simulink model "VehicleModel"  (R2016b)
settings: Solver=FixedStepAuto  StartTime=0.0  StopTime=t_EndSimulation  FixedStep=base_dT  MaxStep=0.01  RelTol=1e-3  EnableMultiTasking=on
values from neighbouring files (symbols this model uses):
  b_E2C_inloop = Simulink.Parameter    [VehicleModelInit.m]
  b_Engine_in_loop = Simulink.Parameter    [VehicleModelInit.m]
  b_initialize_distance_t_startsim = Simulink.Parameter    [VehicleModelInit.m]
  b_Ne_in_loop = Simulink.Parameter    [VehicleModelInit.m]
  b_TTB_in_loop = Simulink.Parameter    [VehicleModelInit.m]
  b_use_acc = Simulink.Parameter    [VehicleModelInit.m]
  b_use_acc_hardset = Simulink.Parameter    [VehicleModelInit.m]
  base_dT = Simulink.Parameter    [VehicleModelInit.m]
  c_acc_d_hdw = Simulink.Parameter    [VehicleModelInit.m]
  c_acc_hdw = Simulink.Parameter    [VehicleModelInit.m]
  c_EngFricCoef = PARS.c_EngFricCoef    [VehicleModelInit.m]
  c_EngFricCoefd = PARS.c_EngFricCoefd    [VehicleModelInit.m]
  d_Ne_max = Simulink.Parameter    [VehicleModelInit.m]
  d_Ne_min = Simulink.Parameter    [VehicleModelInit.m]
  Driver_TuneG1 = PARS.Driver_TuneG1    [VehicleModelInit.m]
  Driver_TuneG2 = PARS.Driver_TuneG2    [VehicleModelInit.m]
  Driver_TuneG3 = PARS.Driver_TuneG3    [VehicleModelInit.m]
  Driver_TuneG_aw = PARS.Driver_TuneG_aw    [VehicleModelInit.m]
  E2C_c2_dTB = Simulink.Parameter    [VehicleModelInit.m]
  E2C_c_dTB = Simulink.Parameter    [VehicleModelInit.m]
  E2C_CycleTimespan = Simulink.Parameter    [VehicleModelInit.m]
  E2C_initializeRelDist = Simulink.Parameter    [VehicleModelInit.m]
  E2C_SpeedShape = Simulink.Parameter    [VehicleModelInit.m]
  E2C_Trap_CycleAcceEndAlpha = Simulink.Parameter    [VehicleModelInit.m]
  E2C_Trap_CycleAcceStartAlpha = Simulink.Parameter    [VehicleModelInit.m]
  E2C_Trap_CycleDeceEndAlpha = Simulink.Parameter    [VehicleModelInit.m]
  E2C_Trap_CycleDeceStartAlpha = Simulink.Parameter    [VehicleModelInit.m]
  E2C_V_High_kmh = Simulink.Parameter    [VehicleModelInit.m]
  E2C_V_Low_kmh = Simulink.Parameter    [VehicleModelInit.m]
  E2C_V_max = Simulink.Parameter    [VehicleModelInit.m]
  E2C_V_min = Simulink.Parameter    [VehicleModelInit.m]
  FTP_speed_1sec = [FTP_speed_once.speed;Idle_speed_once;FTP_speed_once.speed;Idle_speed_once;FTP_speed_once.speed]    [VehicleModelInit.m]
  mass = 3123*1.3    (= 4059.9)    [VehicleModelInit.m]
  T_ACC_TuneG1_data = Simulink.Parameter    [VehicleModelInit.m]
  T_ACC_TuneG1_pt = Simulink.Parameter    [VehicleModelInit.m]
  T_ACC_TuneG2_data = Simulink.Parameter    [VehicleModelInit.m]
  T_ACC_TuneG2_pt = Simulink.Parameter    [VehicleModelInit.m]
  t_StartSimulation = Simulink.Parameter    [VehicleModelInit.m]
  T_TB_ego_ini = Simulink.Parameter    [VehicleModelInit.m]
  T_TB_OffSet = Simulink.Parameter    [VehicleModelInit.m]
  tau_EngTorque = Simulink.Parameter    [VehicleModelInit.m]
  tau_Ne = Simulink.Parameter    [VehicleModelInit.m]
  tau_pedal_dem = Simulink.Parameter    [VehicleModelInit.m]
  VESP_MD = x0.VESP    [VehicleModelInit.m]
undefined symbols (not defined in the file or in its folder): Continuous, DiscIntNeverNeededParam, initializeRelDist, p_ego_ini, p_lead_ini, PedalMapMD, r_w, Simulation_dT, spsSampleAndHoldModel, v_lead_ini, x0
libraries: simulink x9, spsEdgeDetectorModel x6, dspsigops x1
(part 3 of 7)

== matlab function VehicleModel/Subsystem/Follower vehicle Subsystem/Follow Vehicle/Engine DYnamics and Torque converter ==
  data: time_now input; time_start input; d_Ne output; Ne_rpm input; VSpeed input; last_gearlevel input; GearLevel input; F_tract output; EngineTorque input; Simulate_EngineTorque input; outspeed output; w_ratio output; last_p_2_f input; last_d_Ne input; c_EngFricCoef parameter; p_1_e output; p_2_e output; GR output; torque_ratio output; p1e_ratio output; c_EngFricCoefd parameter
% function [d_Ne, F_tract, outspeed, w_ratio] = gearbox_control(time_now, time_start, Ne_rpm, VSpeed, last_gearlevel, GearLevel, EngineTorque, Simulate_EngineTorque, last_p_2_f, c_EngFricCoef)
% function [d_Ne,F_tract,outspeed,w_ratio]  = gearbox_control(Ne_rpm, VSpeed, GearLevel, EngineTorque)
% %#codegen[d_Ne,F_tract,outspeed,w_ratio]
% % Ne_rpm [rpm]
% % VSpeed [m/s]
% % GearLevel [1~6]
% % EngineTorque [Nm]
% % F_tract [N]
% % d_Ne [rpm]
% % d_Ne [rpm]
% p1.e =0;
% p2.e =0;
% p1.f =0;
% p2.f =0;
% % parameters:
% gearRatio = [3.97	2.31	1.51	1.14	0.85	0.67]';
% FR = 3.51;  % checked with Rasoul 0802
% Rw      = 0.41;     % Tire radius [m] changed  % to match engine speed during 200-300s
% effi_trnsmtn = 0.9;  % not the same as before
% J_Eng = 1.53; %  guess. [kg*m^2]
% 
% GR = gearRatio(GearLevel);  
% 
% % ??????? rpm or rad/s?
% % p1.f = Ne_rpm;  % rpm
% % p2.f = VSpeed * 60/2/pi * FR * GR / Rw;  % rpm
% 
% p1.f = 2*pi/60 * Ne_rpm;  % rad/s
% p2.f = VSpeed * FR * GR / Rw;  % rad/s
% 
% 
% 
% if p1.f==0
%     w_ratio = p2.f/0.1;
% else
%     w_ratio = p2.f/p1.f;
% end
% 
% %  convert speed ratio to capacity factor
% thresh1 = 0.99;
% thresh2 = 1.07;
% thresh3 = 0.85;
% a1 = 11;
% a2 = -10.4038;
% a3 = -1.2657862;
% a4 = 0.28137862;
% a5 = 30.9091;
% a6 = 11118.1;
% a7 = 7.22274;
% a8 = -1.10485;
% a9 = -0.102677;
% b1 = 2.1  ;
% b2 = 1.30588 ;
% b3 = 0.99;
% 
% if (w_ratio < thresh1) 
%     kappa = ((a1 + a2 * w_ratio) / (1 + a3 * w_ratio + a4 * w_ratio^2));
% else
%     if (w_ratio < thresh2) 
%         kappa = (a5 + (w_ratio-thresh1)*a6);
%     else
%         kappa = (a7 / (1 + a8 * exp(a9 * w_ratio)));
%     end
% end
% 
% %  convert speed ratio to torque ratio
% if (w_ratio < thresh3) 
%     torque_ratio = (b1 - b2 * w_ratio);
% else
%     torque_ratio = b3;
% end                                                      
%     kappa = kappa/2; % tune the parameters
%     
% 	p1.e = (p1.f/kappa)^2*sign(1-w_ratio);
% 	p2.e = torque_ratio*p1.e;
%     
%     F_tract = p2.e * effi_trnsmtn * GR * FR / Rw; 
% outspeed = p2.f;
%     % EngineTorque - p1.e = J_Eng * d_w_Eng
%     d_Ne = (EngineTorque - p1.e)/J_Eng * 60/2/pi;
% %     if EngineTorque>100
% %         [EngineTorque, p1.e]
% %     end
% end
%%%%%%%%%%%%%%%%%%%%%%%%%%%%%%%%%%%%%%%%%%%%%%%%%

% 
% 
% function [d_Ne,F_tract,outspeed,w_ratio]  = gearbox_control(Ne_rpm, VSpeed, GearLevel, EngineTorque)
% %#codegen
% % Ne_rpm [rpm]
% % VSpeed [m/s]
% % GearLevel [1~6]
% % EngineTorque [Nm]
% % F_tract [N]
% % d_Ne [rpm]
% p1.e =0;
% p2.e =0;
% p1.f =0;
% p2.f =0;
% 
% 
% % parameters:
% gearRatio = [3.97	2.31	1.51	1.14	0.85	0.67]';
% FR = 3.51;  % checked with Rasoul 0802
% Rw      = 0.41;     % Tire radius [m] changed  % to match engine speed during 200-300s
% effi_trnsmtn = 0.9;
% J_Eng = 1.53; %  guess. [kg*m^2]
% 
% GR = gearRatio(GearLevel);  
% 
% % ??????? rpm or rad/s?
% p1.f = Ne_rpm;  % rpm
% p2.f = VSpeed * 60/2/pi * FR * GR / Rw;  % rpm
% 
% p1.f = 2*pi/60 * Ne_rpm;  % rad/s
% p2.f = VSpeed * FR * GR / Rw;  % rad/s
% 
% 
% 
% if p1.f==0
%     w_ratio = p2.f/0.1;
% else
%     w_ratio = p2.f/p1.f;
% end;
% 
% %  convert speed ratio to capacity factor
% % Original Tulga and Xinyi's parameters
% % thresh1 = 0.99;
% % thresh2 = 1.07;
% % thresh3 = 0.85;
% % a1 = 11;
% % a2 = -10.4038;
% % a25 = 0;
% % a3 = -1.2657862;
% % a4 = 0.28137862;
% % a5 = 30.9091;
% % a6 = 11118.1;
% % a7 = 7.22274;
% % a8 = -1.10485;
% % a9 = -0.102677;
% % b1 = 2.1;
% % b2 = 1.30588;
% % b3 = 0.99;
% % TuneRatio = 1;
% 
% % parameters from shape in reference:
% % Nonlinear Robust Control of Torque Converter
% % Clutch Slip System for Passenger Vehicles Using
% % Advanced Torque Estimation Algorithms
% thresh1 = 1;
% thresh2 = 1.07;
% thresh3 = 0.85;
% a1 = 11;
% a2 = -10.4038/1.2;
% a25 = 0;
% a3 = -1.2657862;
% a4 = 0.28137862;
% a5 = 30.9091/43*202;
% a6 = 11118.1;
% a7 = 7.22274*150*2.5/9;
% a8 = -1.10485;
% a9 = -0.102677*4.5;
% b1 = 2.1;
% b2 = 1.30588;
% b3 = 0.99;
% 
% 
% TuneRatio = 2;
% 
% if (w_ratio < thresh1) 
%     kappa = ((a1 + a2 * w_ratio + a25* w_ratio^2) /(1 + a3 * w_ratio + a4 * w_ratio^2));
% else
%     if (w_ratio < thresh2) 
%         kappa = (a5 + (w_ratio-thresh1)*a6);
%     else
%         kappa = 1/sqrt((1/11^2-1/923^2)/4/(1.5-1.07)*(w_ratio-thresh2)+1/923^2);
%         % kappa = (a7 / (1 + a8 * exp(a9 * w_ratio)));
%     end
% end
% kappa = kappa/TuneRatio; % tune the parameters
% %  convert speed ratio to torque ratio
% % 	if (w_ratio < thresh3) 
% % 		torque_ratio = (b1 - b2 * w_ratio);
% % 	else
% % 		torque_ratio = b3;
% %     end                                                     
%     if (w_ratio < thresh3) 
%         torque_ratio = (b1 - b2 * w_ratio);
%     elseif w_ratio >= thresh3 && w_ratio<=1
%         torque_ratio = b3;
%     else
%         torque_ratio = b3 + w_ratio-1;
%     end
% 	p1.e = (p1.f/kappa)^2*sign(1-w_ratio);
% 	p2.e = torque_ratio*p1.e;
%     
%     F_tract = p2.e * effi_trnsmtn * GR * FR / Rw; 
% 
%     % EngineTorque - p1.e = J_Eng * d_w_Eng
%     d_Ne = (EngineTorque - p1.e)/J_Eng * 60/2/pi;
% outspeed = p2.f;
% end
% % 

% %%%%%%%%%%%%%%%%%%%%%%%%%%%%%%%%%%%%%%%%%%%%%%%%%%%%%%
% My original TC:
function [d_Ne,F_tract,outspeed,w_ratio,p_1_e,p_2_e,GR,torque_ratio, p1e_ratio]  = gearbox_control(time_now, time_start, Ne_rpm, VSpeed, last_gearlevel, GearLevel, EngineTorque, Simulate_EngineTorque, last_p_2_f, last_d_Ne, c_EngFricCoef,c_EngFricCoefd)
%#codegen
% Ne_rpm [rpm]
% VSpeed [m/s]
% GearLevel [1~6]
% EngineTorque [Nm]
% F_tract [N]
% d_Ne [rpm]
p1.e =0;
p2.e =0;
p1.f =0;
p2.f =0;


    % parameters:
    gearRatio = [3.97	2.31	1.51	1.14	0.85	0.67]';
    FR = 3.51;  % checked with Rasoul 0802
    Rw      = 0.41;     % Tire radius [m] changed  % to match engine speed during 200-300s
    effi_trnsmtn = 0.9;
    J_Eng = 2.53; % Original value when doing alpha openloop: 1.53; %  guess. [kg*m^2]
    time_duration = [0.7,0.7,0.6,0.5,0.5,0.5] + 0.4;   % 0.5 [s] gear shift duration.
 
    % ---------------------------------------------
    % This part modified based on Tulga's code:
    % ng = gr2 + ((gr1-gr2)/dur)*(time-ts);
    % nt = gr2*eff2 + ((gr1*eff1-gr2*eff2)/dur)*(time-ts);
    
    if time_now < time_start + time_duration(GearLevel)
        ratio = (time_now - time_start)/time_duration(GearLevel);
        GR = gearRatio(GearLevel) * ratio + gearRatio(last_gearlevel) * (1 - ratio);  
        % EngineTorque = Simulate_EngineTorque;  % During shifts, use simulated torque. 
    else
        GR = gearRatio(GearLevel);
    end
    % ---------------------------------------------

    % ??????? rpm or rad/s?
    p1.f = Ne_rpm;  % rpm
    p2.f = VSpeed * 60/2/pi * FR * GR / Rw;  % rpm

    p1.f = 2*pi/60 * Ne_rpm;  % rad/s
    p2.f = VSpeed * FR * GR / Rw;  % rad/s
    % p2.f = max(min(p2.f, last_p_2_f+80*0.02), last_p_2_f-80*0.02); % Removed
    % because already done the smoothing in GR. This line generates similar Ne
    % and slightly less torque than if using linear combination above. 


    if p1.f<=0.1
        w_ratio = p2.f/0.1;
    else
        w_ratio = p2.f/p1.f;
    end
    
    clutch_efficiency = 1;
%     if time_now < time_start + time_duration(GearLevel)
%         clutch_efficiency = w_ratio;
%     else
%         clutch_efficiency = 1;
%     end
    
    %  convert speed ratio to capacity factor

    thresh1 = 1;
    thresh2 = 1.07;
    thresh3 = 0.85;
    a1 = 11.5;
    a2 = -10.4038/1.2;
    a25 = -0.04;
    a3 = -1.2657862;
    a4 = 0.28137862;
    a5 = 30.9091/43*202;
    a6 = 11118.1;
    a7 = 7.22274*150*2.5/9;
    a8 = -1.10485;
    a9 = -0.102677*4.5;
    b1 = 2.1*1.2; % 2.0; % *0.7
    b2 = 1.8; % 3.7765; % 2.5412; % 2.0471; % 1.30588; % 0.5647; % 1.30588 * 0.7;
    b3 = 0.99;
    TuneRatio =2;

% b1 = 1.6;
% b2 = 0.90588;

    if (w_ratio <= thresh1) 
        if  w_ratio >0.5
            % xx=interp1([0.5,0.6,0.7,0.8,0.9,1],[0.9,0.85,0.7,0.6,0.3,0.01],w_ratio,'PCHIP');
            xx=interp1([0.5,0.6,0.7,0.8,0.9,1],[0.85,0.78,0.65,0.5,0.3,0.01],w_ratio,'PCHIP');
            xx = max(xx,0);
            kappa = sqrt(1/xx/0.033)*TuneRatio;

        else
            % xx=interp1([0,0.4,0.5],[1,0.95,0.9],w_ratio,'PCHIP');
            xx=interp1([0,0.4,0.5],[1,0.9,0.85],w_ratio,'PCHIP');
            xx = max(xx,0);
            kappa = sqrt(1/xx/0.033)*TuneRatio;

        end
    else
        if (w_ratio < thresh2) 
            kappa = (a5 + (w_ratio-thresh1)*a6);
        else
            kappa = (1/sqrt((1/11^2-1/923^2)/4/(1.5-1.07)*(w_ratio-thresh2)+1/923^2))*1.0;
            % kappa = ((a7+(exp(w_ratio))^-2-2) / (1 + a8 * exp(a9 * w_ratio)))+1/(10^20*(25*(w_ratio-thresh2)+0.1).^20);
        end
    end

    if (w_ratio < thresh3) 
        torque_ratio = (b1 - b2 * w_ratio);
    elseif (w_ratio >= thresh3) && (w_ratio<=1)
        torque_ratio = b3;
    else
        % torque_ratio = b3 + (w_ratio-1)*2;
        torque_ratio = b3 + (w_ratio-1)*1 + 2*((1-1.5)^2-(w_ratio-1.5)^2);
        % torque_ratio = b3;
        % torque_ratio = b3 + w_ratio-1;
    end
    kappa = kappa/TuneRatio; % tune the parameters

	p1.e = (p1.f/kappa)^2*sign(1-w_ratio);
	p2.e = torque_ratio*p1.e * clutch_efficiency;
    
    F_tract = p2.e * effi_trnsmtn * GR * FR / Rw; 

    % EngineTorque - p1.e = J_Eng * d_w_Eng
    
    d_Ne = (EngineTorque - p1.e - c_EngFricCoef*(Ne_rpm-500) - c_EngFricCoefd*last_d_Ne)/J_Eng * 60/2/pi;
    
    p_1_e = p1.e;
    p_2_e = p2.e;
    
    outspeed = p2.f;
    p1e_ratio = 1/(kappa)^2;
    
end

%%%%%%%%%%%%%%%%%%%%%%%%%%%%%%%%%%%%%%%%%%
% Try Tulga's torque converter
% 
% 
% function [d_Ne,F_tract,outspeed,w_ratio]  = gearbox_control(...
% time_now, time_start, Ne_rpm, VSpeed, last_gearlevel, GearLevel, ...
%     EngineTorque, Simulate_EngineTorque, last_p_2_f, c_EngFricCoef)
%     % Ne_rpm, VSpeed, GearLevel, EngineTorque)
% 
% %#codegen
% % Ne_rpm [rpm]
% % VSpeed [m/s]
% % GearLevel [1~6]
% % EngineTorque [Nm]
% % F_tract [N]
% % d_Ne [rpm]
% p1.e =0;
% p2.e =0;
% p1.f =0;
% p2.f =0;
% 
% 
% % parameters:
% gearRatio = [3.97	2.31	1.51	1.14	0.85	0.67]';
% FR = 3.51;  % checked with Rasoul 0802
% Rw      = 0.41;     % Tire radius [m] changed  % to match engine speed during 200-300s
% effi_trnsmtn = 0.9;
% J_Eng = 1.53; %  guess. [kg*m^2]
% time_duration = [0.7,0.7,0.6,0.5,0.5,0.5] + 0.2;   % 0.5 [s] gear shift duration.
% 
% % GR = gearRatio(GearLevel);  
% if time_now < time_start + time_duration(GearLevel)
%     ratio = (time_now - time_start)/time_duration(GearLevel);
%     GR = gearRatio(GearLevel) * ratio + gearRatio(last_gearlevel) * (1 - ratio);  
%     % EngineTorque = Simulate_EngineTorque;  % During shifts, use simulated torque. 
% else
%     GR = gearRatio(GearLevel);
% end
% 
% 
% % ??????? rpm or rad/s?
% p1.f = Ne_rpm;  % rpm
% p2.f = VSpeed * 60/2/pi * FR * GR / Rw;  % rpm
% 
% p1.f = 2*pi/60 * Ne_rpm;  % rad/s
% p2.f = VSpeed * FR * GR / Rw;  % rad/s
% 
% 
% 
% if p1.f==0
%     w_ratio = p2.f/0.1;
% else
%     w_ratio = p2.f/p1.f;
% end;
% 
% % %  convert speed ratio to capacity factor
% % % Original Tulga and Xinyi's parameters
% % thresh1 = 0.99;
% % thresh2 = 1.07;
% % thresh3 = 0.85;
% % a1 = 11;
% % a2 = -10.4038;
% % a25 = 0;
% % a3 = -1.2657862;
% % a4 = 0.28137862;
% % a5 = 30.9091;
% % a6 = 11118.1;
% % a7 = 7.22274;
% % a8 = -1.10485;
% % a9 = -0.102677;
% % b1 = 2.1;
% % b2 = 1.30588;
% % b3 = 0.99;
% % TuneRatio = 1;
% 
% % parameters from shape in reference:
% % Nonlinear Robust Control of Torque Converter
% % Clutch Slip System for Passenger Vehicles Using
% % Advanced Torque Estimation Algorithms
% thresh1 = 1;
% thresh2 = 1.07;
% thresh3 = 0.85;
% a1 = 11;
% a2 = -10.4038/1.2;
% a25 = 0;
% a3 = -1.2657862;
% a4 = 0.28137862;
% a5 = 30.9091/43*202;
% a6 = 11118.1;
% a7 = 7.22274*150*2.5/9;
% a8 = -1.10485;
% a9 = -0.102677*4.5;
% b1 = 2.1;
% b2 = 1.30588;
% b3 = 0.99;
% % 
% % 
% TuneRatio = 2;
% 
% if (w_ratio < thresh1) 
%     kappa = ((a1 + a2 * w_ratio + a25* w_ratio^2) /(1 + a3 * w_ratio + a4 * w_ratio^2));
% else
%     if (w_ratio < thresh2) 
%         kappa = (a5 + (w_ratio-thresh1)*a6);
%     else
%         kappa = 1/sqrt((1/11^2-1/923^2)/4/(1.5-1.07)*(w_ratio-thresh2)+1/923^2);
%         % kappa = (a7 / (1 + a8 * exp(a9 * w_ratio)));
%     end
% end
% kappa = kappa/TuneRatio; % tune the parameters
% %  convert speed ratio to torque ratio
% % 	if (w_ratio < thresh3) 
% % 		torque_ratio = (b1 - b2 * w_ratio);
% % 	else
% % 		torque_ratio = b3;
% %     end                                                     
%     if (w_ratio < thresh3) 
%         torque_ratio = (b1 - b2 * w_ratio);
%     elseif w_ratio >= thresh3 && w_ratio<=1
%         torque_ratio = b3;
%     else
%         torque_ratio = b3 + w_ratio-1;
%     end
% 	p1.e = (p1.f/kappa)^2*sign(1-w_ratio);
% 	p2.e = torque_ratio*p1.e;
%     
%     F_tract = p2.e * effi_trnsmtn * GR * FR / Rw; 
% 
%     % EngineTorque - p1.e = J_Eng * d_w_Eng
%     d_Ne = (EngineTorque - p1.e)/J_Eng * 60/2/pi;
% outspeed = p2.f;
% end
% %

== matlab function VehicleModel/Subsystem/Follower vehicle Subsystem/Follow Vehicle/PthsetTq model ==
  data: Tq_vec output; Ne_vec input; Torque_vec input; VSpeed_vec input
function Tq_vec    = PthsetModel(Ne_vec, Torque_vec, VSpeed_vec)
%#codegen


FordTqCal.Ne = [500;500;500;500;500;500;500;500;600;600;600;600;600;600;600;600;800;800;800;800;800;800;800;800;800;1000;1000;1000;1000;1000;1000;1000;1000;1000;1000;1200;1200;1200;1200;1200;1200;1200;1200;1200;1200;1200;1400;1400;1400;1400;1400;1400;1400;1400;1400;1400;1400;1400;1400;1400;1600;1600;1600;1600;1600;1600;1600;1600;1600;1600;1600;1600;1600;1600;1600;1600;1800;1800;1800;1800;1800;1800;1800;1800;1800;1800;1800;1800;1800;1800;1800;1800;1800;2000;2000;2000;2000;2000;2000;2000;2000;2000;2000;2000;2000;2000;2000;2000;2000;2000;2200;2200;2200;2200;2200;2200;2200;2200;2200;2200;2200;2200;2200;2200;2200;2200;2200;2400;2400;2400;2400;2400;2400;2400;2400;2400;2400;2400;2400;2400;2400;2400;2400;2400;2600;2600;2600;2600;2600;2600;2600;2600;2600;2600;2600;2600;2600;2600;2600;2600;2600;2800;2800;2800;2800;2800;2800;2800;2800;2800;2800;2800;2800;2800;2800;2800;2800;2800;3000;3000;3000;3000;3000;3000;3000;3000;3000;3000;3000;3000;3000;3000;3000;3000;3200;3200;3200;3200;3200;3200;3200;3200;3200;3200;3200;3200;3200;3200;3200;3400;3400;3400;3400;3400;3400;3400;3400;3400;3400;3400;3400;3400;500;600;800;1000;1200;1400;1600;1800;2000;2200;2400;2600;2800;3000;3200;3400];
FordTqCal.Torque = [-74.9710029200000;-16.8452928900000;22.5768412100000;66.3118405400000;122.485125100000;171.724968200000;209.291492900000;327.216453100000;-69.7798932200000;-17.2465227700000;24.2147953500000;71.9971179100000;108.756652100000;165.981760000000;232.925894200000;339.093048300000;-71.2481971900000;6.78186051200000;38.9692268100000;99.4179257300000;149.909041800000;196.908789400000;242.879963800000;344.770267100000;422.698119600000;-77.1395675800000;2.25202763800000;42.2012448800000;93.5939964800000;136.909750000000;186.449928000000;240.720366800000;341.467734600000;436.725202700000;518.667213700000;-77.8024739700000;-3.56634450800000;41.4527193700000;93.4652855300000;142.232771000000;187.634317800000;236.637760000000;333.810753400000;431.126064600000;524.171115900000;615.577708700000;-83.4754614100000;-8.34883757200000;37.4277251100000;92.8230069100000;140.027350900000;182.326160900000;231.941433200000;328.194558900000;424.562740900000;511.984434000000;616.532564800000;717.468056700000;811.174744000000;854.007744200000;-94.0440471900000;-11.9160323900000;33.5026669500000;81.9477706700000;136.063332400000;181.688248000000;229.433752100000;327.668074700000;421.229442600000;505.624945100000;607.627890900000;702.803483900000;796.506491400000;901.631690000000;1006.15607900000;1167.16171800000;-105.810334300000;-29.5507777900000;26.4565543900000;79.4188075700000;129.112641000000;174.814601000000;227.881676400000;320.856473100000;409.287739500000;498.839210100000;595.698470400000;692.151257500000;782.649266900000;879.386444600000;991.660780600000;1084.17976600000;1166.69977800000;-115.283222900000;-26.7879707200000;30.5205674100000;71.0457994800000;115.255625000000;163.862045400000;213.681720400000;312.680641600000;402.357125500000;491.118597900000;585.701714300000;684.640373900000;777.887954900000;871.133695900000;978.600076500000;1069.07187300000;1159.94140700000;-117.321614400000;-35.7200974500000;13.9601127100000;65.4809546500000;107.970297900000;157.171490300000;206.297887200000;308.097810300000;387.385807300000;489.362517700000;575.402137900000;676.483194500000;768.282516600000;857.450964200000;959.454329600000;1055.35717600000;1161.03658800000;-124.259281100000;-43.0894697100000;9.89302132700000;59.3682431900000;99.0452310000000;149.131037800000;197.173036500000;296.308032200000;373.776023900000;471.134821700000;565.528338100000;659.058943700000;749.259571300000;843.445347900000;945.856414300000;1036.61175100000;1159.60480900000;-135.365963400000;-61.2876489400000;-4.33545738900000;41.0434879000000;90.6662490300000;137.731564000000;186.322276200000;279.595050000000;364.630774700000;457.697283200000;551.990748200000;640.398723700000;730.372979000000;818.138407600000;919.270429500000;1012.50988300000;1144.92866700000;-154.608877100000;-62.4754987700000;-13.0688869200000;35.1175674200000;78.5403251000000;131.062560100000;176.973940900000;267.098275700000;355.041255000000;439.823605800000;530.465621200000;615.923600900000;700.034455300000;789.041537900000;888.954149400000;980.416288500000;1117.56934700000;-166.473853800000;-95.8158145100000;-30.2112397100000;20.7283938700000;66.7200572800000;113.495783000000;162.476945100000;258.772843200000;342.012303800000;426.753454600000;521.939682100000;602.320677600000;682.204738400000;762.344949700000;873.583209600000;992.218131200000;-173.479879900000;-101.615500000000;-50.5548781900000;5.59668278300000;48.8622091200000;99.0922829400000;147.984848200000;232.803380700000;327.097768100000;400.176971300000;486.274910900000;575.903432100000;672.200276300000;766.611653100000;813.925270700000;-177.160793600000;-110.511019900000;-63.6365230300000;-14.9158481100000;30.4639121500000;78.5632367300000;129.668192000000;224.303438100000;301.548553800000;389.638590300000;473.171130000000;566.041266600000;638.739388800000;-1000;-1000;-1000;-1000;-1000;-1000;-1000;-1000;-1000;-1000;-1000;-1000;-1000;-1000;-1000;-1000];
FordTqCal.PthsetTq = [0;50;100;150;200;250;300;400;0;50;100;150;200;250;300;400;0;50;100;150;200;250;300;400;500;0;50;100;150;200;250;300;400;500;600;0;50;100;150;200;250;300;400;500;600;700;0;50;100;150;200;250;300;400;500;600;700;800;900;1000;0;50;100;150;200;250;300;400;500;600;700;800;900;1000;1100;1300;0;50;100;150;200;250;300;400;500;600;700;800;900;1000;1100;1200;1300;0;50;100;150;200;250;300;400;500;600;700;800;900;1000;1100;1200;1300;0;50;100;150;200;250;300;400;500;600;700;800;900;1000;1100;1200;1300;0;50;100;150;200;250;300;400;500;600;700;800;900;1000;1100;1200;1350;0;50;100;150;200;250;300;400;500;600;700;800;900;1000;1100;1200;1350;0;50;100;150;200;250;300;400;500;600;700;800;900;1000;1100;1200;1350;0;50;100;150;200;250;300;400;500;600;700;800;900;1000;1100;1250;0;50;100;150;200;250;300;400;500;600;700;800;900;1000;1050;0;50;100;150;200;250;300;400;500;600;700;800;850;0;0;0;0;0;0;0;0;0;0;0;0;0;0;0;0];

Tq_vec = griddata(FordTqCal.Ne, FordTqCal.Torque, FordTqCal.PthsetTq, Ne_vec, Torque_vec);
Tq_vec( intersect(find(VSpeed_vec<2), find(Torque_vec<5) )) = 150;
Tq_vec( intersect( find(isnan(Tq_vec)), find(Torque_vec<0)) )=0;

== matlab function VehicleModel/Subsystem/Follower vehicle Subsystem/Follow Vehicle/Engine model1 ==
  data: engineoutNOx_ppm output; Ne_vec input; Tq_vec input; meu_kg_s output
function [engineoutNOx_ppm, meu_kg_s]      = EngineModel(Ne_vec, Tq_vec)
%#codegen
FordData.C_NOx_eu=[2.25762409700000,1.48625333300000,2.53227143100000,1.40526886500000,1.48376886900000,1.08211845400000,1.22896117600000,0.774905453000000,1.43134235500000,1.10964119300000,1.16812440600000,0.912941239000000,1.27689041400000,0.840189182000000,1.68537425400000,1.06896694300000;77.7336189200000,66.7131323400000,83.1490420600000,71.4323197300000,78.6699699800000,83.1126174900000,91.0357459700000,80.5169999300000,86.1282940600000,74.9800580500000,77.9368165100000,67.3535086200000,67.6916369000000,52.9319036300000,57.6801792200000,56.9409641600000;93.4701856100000,73.0093723900000,93.1112276200000,63.5327023300000,70.5283689500000,69.8944052300000,69.7843775900000,78.9711420600000,108.102874500000,99.0763243400000,109.785688800000,103.569999900000,111.936107900000,108.116904900000,138.463511700000,161.283675000000;115.900969600000,98.1385357700000,90.1779151700000,75.7649708100000,68.3221778600000,61.6508764000000,80.9472557300000,92.3232953600000,118.429404700000,118.138823600000,125.300058600000,131.164566000000,147.137470100000,152.844180100000,218.902575100000,277.520714200000;244.974877800000,208.876505900000,132.824970000000,97.4586493500000,78.8352280100000,77.3417367800000,108.319940000000,113.631075200000,131.433696700000,141.663772500000,139.357590500000,161.691976400000,176.291578900000,192.054131800000,282.689702500000,409.127621500000;611.801796900000,455.626928300000,203.786423900000,135.014024300000,114.974255700000,105.941999700000,128.123614400000,139.780695500000,174.086505800000,179.955149700000,192.886726200000,211.508862200000,235.443617300000,238.055294500000,360.565449900000,547.683923500000;1331.45555700000,1219.17445500000,456.065104100000,220.679940100000,134.895568700000,124.843727900000,157.453367900000,179.159511200000,246.544523800000,254.239942600000,278.443091200000,283.519117800000,302.382694400000,297.501244000000,453.310748900000,678.719456500000;1689.28144100000,1662.56946000000,1809.85647000000,756.339463100000,279.077382200000,175.138930500000,189.261489800000,223.400363300000,291.671666000000,349.664945600000,388.014190700000,413.407484800000,433.835298400000,420.357427800000,608.756011200000,876.977261900000;1689.28144100000,1662.56946000000,2030.22882400000,2372.79262800000,604.193954500000,305.600904600000,261.407409900000,262.680665700000,349.460689000000,508.980239700000,542.334583100000,560.582959100000,544.666544600000,596.865821800000,773.404254300000,950.574495400000;1689.28144100000,1662.56946000000,2030.22882400000,1903.18924700000,1065.21376900000,549.108273800000,462.245157500000,361.353571400000,486.090349200000,651.363421300000,655.258364400000,676.150537900000,615.765239500000,686.080323600000,847.960568400000,1032.08809900000;1689.28144100000,1662.56946000000,2030.22882400000,1903.18924700000,1838.81377000000,1293.62411500000,766.547606300000,634.774793300000,700.457916600000,738.703189700000,735.874044500000,728.241260300000,678.368811500000,715.053387000000,881.818869800000,1066.88343700000;1689.28144100000,1662.56946000000,2030.22882400000,1903.18924700000,1838.81377000000,1698.37125200000,1142.32010400000,964.476765700000,940.581138700000,877.995809400000,851.089467800000,793.700416400000,780.098073200000,795.836746800000,934.802528500000,1059.46738200000;1689.28144100000,1662.56946000000,2030.22882400000,1903.18924700000,1838.81377000000,1869.57849400000,1747.34970100000,1358.95454200000,1138.71021400000,915.954867900000,899.966250500000,897.467100600000,866.129469200000,837.367378600000,920.021667500000,1031.69091400000;1689.28144100000,1662.56946000000,2030.22882400000,1903.18924700000,1838.81377000000,1759.27605400000,1998.77750900000,1517.83313700000,1276.92765800000,1054.38757200000,908.992011100000,922.976109300000,904.774372800000,833.394516900000,892.743814300000,1031.69091400000;1689.28144100000,1662.56946000000,2030.22882400000,1903.18924700000,1838.81377000000,1759.27605400000,1936.27559700000,1736.12530100000,1538.87784600000,1259.82010600000,1122.27134200000,1040.75706100000,997.544178500000,902.754910600000,897.219403800000,1031.69091400000;1689.28144100000,1662.56946000000,2030.22882400000,1903.18924700000,1838.81377000000,1759.27605400000,1643.64035700000,1776.66432900000,1639.86910900000,1405.51736700000,1269.69058700000,1111.13832700000,979.684554000000,899.367364400000,897.219403800000,1031.69091400000;1689.28144100000,1662.56946000000,2030.22882400000,1903.18924700000,1838.81377000000,1759.27605400000,1643.64035700000,1677.73846200000,1572.58036400000,1358.57810700000,1204.91369200000,1046.82235300000,882.208603300000,899.367364400000,897.219403800000,1031.69091400000];
FordData.spd=[500,600,800,1000,1200,1400,1600,1800,2000,2200,2400,2600,2800,3000,3200,3400;500,600,800,1000,1200,1400,1600,1800,2000,2200,2400,2600,2800,3000,3200,3400;500,600,800,1000,1200,1400,1600,1800,2000,2200,2400,2600,2800,3000,3200,3400;500,600,800,1000,1200,1400,1600,1800,2000,2200,2400,2600,2800,3000,3200,3400;500,600,800,1000,1200,1400,1600,1800,2000,2200,2400,2600,2800,3000,3200,3400;500,600,800,1000,1200,1400,1600,1800,2000,2200,2400,2600,2800,3000,3200,3400;500,600,800,1000,1200,1400,1600,1800,2000,2200,2400,2600,2800,3000,3200,3400;500,600,800,1000,1200,1400,1600,1800,2000,2200,2400,2600,2800,3000,3200,3400;500,600,800,1000,1200,1400,1600,1800,2000,2200,2400,2600,2800,3000,3200,3400;500,600,800,1000,1200,1400,1600,1800,2000,2200,2400,2600,2800,3000,3200,3400;500,600,800,1000,1200,1400,1600,1800,2000,2200,2400,2600,2800,3000,3200,3400;500,600,800,1000,1200,1400,1600,1800,2000,2200,2400,2600,2800,3000,3200,3400;500,600,800,1000,1200,1400,1600,1800,2000,2200,2400,2600,2800,3000,3200,3400;500,600,800,1000,1200,1400,1600,1800,2000,2200,2400,2600,2800,3000,3200,3400;500,600,800,1000,1200,1400,1600,1800,2000,2200,2400,2600,2800,3000,3200,3400;500,600,800,1000,1200,1400,1600,1800,2000,2200,2400,2600,2800,3000,3200,3400;500,600,800,1000,1200,1400,1600,1800,2000,2200,2400,2600,2800,3000,3200,3400];
FordData.tq=[0,0,0,0,0,0,0,0,0,0,0,0,0,0,0,0;50,50,50,50,50,50,50,50,50,50,50,50,50,50,50,50;100,100,100,100,100,100,100,100,100,100,100,100,100,100,100,100;150,150,150,150,150,150,150,150,150,150,150,150,150,150,150,150;200,200,200,200,200,200,200,200,200,200,200,200,200,200,200,200;250,250,250,250,250,250,250,250,250,250,250,250,250,250,250,250;300,300,300,300,300,300,300,300,300,300,300,300,300,300,300,300;400,400,400,400,400,400,400,400,400,400,400,400,400,400,400,400;500,500,500,500,500,500,500,500,500,500,500,500,500,500,500,500;600,600,600,600,600,600,600,600,600,600,600,600,600,600,600,600;700,700,700,700,700,700,700,700,700,700,700,700,700,700,700,700;800,800,800,800,800,800,800,800,800,800,800,800,800,800,800,800;900,900,900,900,900,900,900,900,900,900,900,900,900,900,900,900;1000,1000,1000,1000,1000,1000,1000,1000,1000,1000,1000,1000,1000,1000,1000,1000;1100,1100,1100,1100,1100,1100,1100,1100,1100,1100,1100,1100,1100,1100,1100,1100;1300,1300,1300,1300,1300,1300,1300,1300,1300,1300,1300,1300,1300,1300,1300,1300;1350,1350,1350,1350,1350,1350,1350,1350,1350,1350,1350,1350,1350,1350,1350,1350];
FordData.mf_exh=[0.0222201161722222,0.0261227567777778,0.0364507511944444,0.0444147394722222,0.0550398765833333,0.0538654870555556,0.0617080297222222,0.0704047941666667,0.0892050230833333,0.0996783075000000,0.115250554166667,0.121955388722222,0.165041477000000,0.172536466027778,0.179802435027778,0.180158609277778;0.0134139469250000,0.0142574858972222,0.0203560368277778,0.0228295075500000,0.0321581553611111,0.0385680183888889,0.0540706550277778,0.0622903021944444,0.0781091206944445,0.0883644611111111,0.102701624222222,0.125067057861111,0.138617233333333,0.194396566777778,0.194360394277778,0.201813565361111;0.0151453645722222,0.0157616901555556,0.0248099178611111,0.0263730004222222,0.0369082367222222,0.0396519276944445,0.0492013194722222,0.0568515790555556,0.0841871218333333,0.0899530240277778,0.112260673666667,0.125144707277778,0.154217175194444,0.173647865222222,0.206997958583333,0.222232479916667;0.0182925148777778,0.0194734982083333,0.0309969207777778,0.0340508131111111,0.0446032621944444,0.0472998726666667,0.0607113672500000,0.0702795629722222,0.0949918824722222,0.104749922944444,0.127110643305556,0.140728745694444,0.173344537083333,0.196093489944444,0.227365939000000,0.238854541777778;0.0238039997805556,0.0249774504916667,0.0379987580000000,0.0416188704444444,0.0568884355555556,0.0609386163611111,0.0847834084444444,0.0896745246111111,0.115521257750000,0.126524634000000,0.148547286583333,0.163671496111111,0.194999011388889,0.212310709277778,0.244906119388889,0.264081846500000;0.0311280099722222,0.0327563324444444,0.0441627721388889,0.0498990351388889,0.0693606662500000,0.0758114927777778,0.100260420916667,0.105970068944444,0.132385313444444,0.140157305222222,0.163293161944444,0.177366220527778,0.211913479111111,0.230291161833333,0.263570475916667,0.281093559166667;0.0351658429444444,0.0403506536111111,0.0552125600000000,0.0580909796944444,0.0775764724166667,0.0900971961388889,0.115584580805556,0.122659488472222,0.147222040972222,0.156230804722222,0.182210699000000,0.194745808722222,0.232062186472222,0.247541714333333,0.284058489444444,0.303019303055556;0.0361172849444444,0.0428523481944444,0.0714628462500000,0.0740483666666667,0.0967477504166667,0.107427697444444,0.139671371500000,0.150201069750000,0.177770662194444,0.191445090194444,0.220594514805556,0.234445567277778,0.265698305166667,0.287176395000000,0.320455326388889,0.343239170277778;0.0361172849444444,0.0428523481944444,0.0714147649166667,0.0988104419722222,0.114507710111111,0.127543810138889,0.160896919805556,0.176268782194444,0.205841057138889,0.222515184750000,0.249454045666667,0.272626872055556,0.307357703333333,0.334507464444444,0.368134304166667,0.381553144722222;0.0361172849444444,0.0428523481944444,0.0714147649166667,0.116060479833333,0.134216002000000,0.150125986333333,0.185002720444444,0.202608397638889,0.235286381944444,0.259915813277778,0.289540104722222,0.317300009444444,0.347370632777778,0.379357033888889,0.406308280555556,0.420501987500000;0.0361172849444444,0.0428523481944444,0.0714147649166667,0.116060479833333,0.152969785944444,0.183525599555556,0.215571163583333,0.236085944833333,0.272239364638889,0.295124365833333,0.327368946666667,0.353606658333333,0.386155454166667,0.420269493055556,0.440178826944444,0.452671332500000;0.0361172849444444,0.0428523481944444,0.0714147649166667,0.116060479833333,0.152969785944444,0.211371425027778,0.238633718694444,0.267008850027778,0.305876973888889,0.331024745833333,0.364053603055556,0.387450258333333,0.426894383055556,0.448956725555556,0.477376410833333,0.487074578055556;0.0361172849444444,0.0428523481944444,0.0714147649166667,0.116060479833333,0.152969785944444,0.241305586472222,0.275142683527778,0.299738912777778,0.339423997777778,0.359594236111111,0.392347168333333,0.423283300277778,0.456106323333333,0.485089576666667,0.509712682500000,0.515900960833333;0.0361172849444444,0.0428523481944444,0.0714147649166667,0.116060479833333,0.152969785944444,0.254946515444444,0.306628584444444,0.327624446666667,0.369276058888889,0.392383280000000,0.424007270555556,0.450823060833333,0.487337205000000,0.512954776666667,0.541410328888889,0.515900960833333;0.0361172849444444,0.0428523481944444,0.0714147649166667,0.116060479833333,0.152969785944444,0.254946515444444,0.327809767222222,0.355514881111111,0.397054853611111,0.422657404444444,0.457619217222222,0.483694314444444,0.524094080555556,0.542386471388889,0.553279756111111,0.515900960833333;0.0361172849444444,0.0428523481944444,0.0714147649166667,0.116060479833333,0.152969785944444,0.254946515444444,0.358302937222222,0.378259473333333,0.421358479166667,0.449955181944444,0.486174160833333,0.512832017777778,0.546534329166667,0.575651193611111,0.553279756111111,0.515900960833333;0.0361172849444444,0.0428523481944444,0.0714147649166667,0.116060479833333,0.152969785944444,0.254946515444444,0.358302937222222,0.401530492222222,0.438417056944444,0.476779187222222,0.517825519722222,0.547435946111111,0.589331641666667,0.575651193611111,0.553279756111111,0.515900960833333];

meu_kg_s = interp2(FordData.spd, FordData.tq, FordData.mf_exh, Ne_vec, Tq_vec);   % exhaust flow rate [kg/s]
engineoutNOx_ppm = interp2(FordData.spd, FordData.tq, FordData.C_NOx_eu, Ne_vec, Tq_vec);  % engine out nox [ppm] 
engineoutNOx_g_s = engineoutNOx_ppm.*meu_kg_s *1e-3*31.6/29;

== matlab function VehicleModel/E2C_model/MATLAB Function ==
  data: t_ input; v_lead output; NP_trial input; RMSE input; Offset input; E2C_SpeedShape input; E2C_CycleTimespan input; v_lead_pre output; E2C_Trap_CycleAcceStartAlpha input; E2C_Trap_CycleAcceEndAlpha input; E2C_Trap_CycleDeceStartAlpha input; E2C_Trap_CycleDeceEndAlpha input; E2C_V_High input; E2C_V_Low input; E2C_V_min input; FTP_Speed input
% function [v_lead,v_lead_pre] = fcn(t_,NP_trial,RMSE,Offset,v_preview_time,v_preview_value)
function [v_lead,v_lead_pre] = fcn(t_,NP_trial,RMSE,Offset,...
    E2C_SpeedShape,...
    E2C_CycleTimespan,E2C_Trap_CycleAcceStartAlpha,E2C_Trap_CycleAcceEndAlpha,E2C_Trap_CycleDeceStartAlpha,...
    E2C_Trap_CycleDeceEndAlpha,E2C_V_High,E2C_V_Low,...
    E2C_V_min,FTP_Speed)

% 
% v_trial = zeros(50,1);
% coder.varsize('v_trial', [50,1]);
% for i = 1:NP_trial
%     v_trial(i) = i;
% end
%% create v_lead_total and time for lead trace: 
v_lead = 0;
v_lead_pre = zeros(41,1);
switch E2C_SpeedShape
    case 0  % constant speed E2C_V_High
        v_lead = (E2C_V_High);
        v_lead_pre = (ones(41,1)*E2C_V_High);
    case 1   % Trapezoid
        v_lead_total = [E2C_V_min;E2C_V_Low;E2C_V_Low;E2C_V_High;E2C_V_High;E2C_V_Low;E2C_V_Low;E2C_V_min];
        time = [0-10;0;E2C_Trap_CycleAcceStartAlpha;E2C_Trap_CycleAcceEndAlpha;...
            E2C_Trap_CycleDeceStartAlpha;E2C_Trap_CycleDeceEndAlpha;1;+10]*E2C_CycleTimespan;
        for i = 1:NP_trial+1
            v_lead_pre(i) = (interp1(time,v_lead_total,rem(t_+i-1, E2C_CycleTimespan))+RMSE*randn(1)+Offset);
        end
        v_lead = v_lead_pre(1);
        
    case 2  % sinuisoid
        v_lead_pre=(E2C_V_High-E2C_V_Low)/2*sin(2*pi*1/E2C_CycleTimespan*((t_)+[0:40]')) + (E2C_V_High+E2C_V_Low)/2;
        v_lead = v_lead_pre(1);
    case 3
%         for i = 1:NP_trial+1
%             v_lead_pre(i) = max(0,interp1([0:1:(length(FTP_Speed)-1)]',FTP_Speed,rem(t_+i-1, length(FTP_Speed)))+RMSE*randn(1)+Offset);
%         end
%         v_lead = v_lead_pre(1);
        
        FTP_Speed_ext = [FTP_Speed;zeros(50,1)];
        for i = 1:NP_trial+1
            v_lead_pre(i) = max(0,interp1([0:1:(length(FTP_Speed_ext)-1)]',FTP_Speed_ext,rem(t_+i-1, length(FTP_Speed_ext)))+RMSE*randn(1)+Offset);
        end
        v_lead = v_lead_pre(1);
        
    otherwise
        v_lead = (E2C_V_High);
        v_lead_pre = (ones(41,1)*E2C_V_High);
end


%%
end

== matlab function VehicleModel/Subsystem/Follower vehicle Subsystem/Follow Vehicle/DRIVER_RSL/idle control ==
  data: is_in_change input; idle_control_prev input; out_alpha output; clutch_new input; Ne_rpm input; speed_mps input; des_speed_mps input; last_des_speed_mps input; last_brake input; brake input; last_alpha input; alpha input; base_dT input; out_brake output; idle_control output
function [out_alpha,out_brake,idle_control]  = fcn(is_in_change, idle_control_prev, clutch_new, Ne_rpm, speed_mps, des_speed_mps, last_des_speed_mps, last_brake, brake, last_alpha, alpha, base_dT)
idle_control = 0;

if is_in_change
    idle_control = idle_control_prev;
else
    if clutch_new == 0
        if idle_control_prev == 0 % not in idle control mode
            if (des_speed_mps < 0.1 && speed_mps < 0.35) && Ne_rpm < 630
                if (last_brake - brake) < 1e-4 && alpha < 1e-4
                    idle_control = 1;    % turn on idle_control
                else
                    idle_control = 0;
                end
            end
        end
        if idle_control_prev == 1 % already in idle control mode
            if ((des_speed_mps < last_des_speed_mps || des_speed_mps<0.01) && speed_mps < 0.35 ) && Ne_rpm < 630
            % if ((des_speed_mps < last_des_speed_mps || des_speed_mps<0.1) && speed_mps < 0.35 ) && Ne_rpm < 630
                idle_control = 1;   % keep idle control mode
            else
                idle_control = 0;
            end
        end
    else
        idle_control = 0;
    end
end

% Turn off idle_control
% idle_control = 0;


if idle_control == 1
    % override the alpha and brake command
    out_alpha = max(min(last_alpha+0.60*base_dT, 0.11), last_alpha-0.60*base_dT);
    % 0.6 is the alpha rate limit
    out_brake = 0.20;
else
    out_alpha = alpha;
    out_brake = brake;
end

== matlab function VehicleModel/Subsystem/Follower vehicle Subsystem/Follow Vehicle/Engine DYnamics and Torque converter_previous commit: 59d14663b7b119b8a1d5fd64e8bda04b6003aa64 ==
  data: time_now input; time_start input; d_Ne output; Ne_rpm input; VSpeed input; last_gearlevel input; GearLevel input; F_tract output; EngineTorque input; outspeed output; w_ratio output; p_1_e output; last_p_2_f input; p_2_e output; GR output; d_Ne_in input
% function [d_Ne,F_tract,outspeed,w_ratio]  = gearbox_control(Ne_rpm, VSpeed, GearLevel, EngineTorque)
% %#codegen[d_Ne,F_tract,outspeed,w_ratio]
% % Ne_rpm [rpm]
% % VSpeed [m/s]
% % GearLevel [1~6]
% % EngineTorque [Nm]
% % F_tract [N]
% % d_Ne [rpm]
% % d_Ne [rpm]
% p1.e =0;
% p2.e =0;
% p1.f =0;
% p2.f =0;
% % parameters:
% gearRatio = [3.97	2.31	1.51	1.14	0.85	0.67]';
% FR = 3.51;  % checked with Rasoul 0802
% Rw      = 0.41;     % Tire radius [m] changed  % to match engine speed during 200-300s
% effi_trnsmtn = 0.9;  % not the same as before
% J_Eng = 1.53; %  guess. [kg*m^2]
% 
% GR = gearRatio(GearLevel);  
% 
% % ??????? rpm or rad/s?
% % p1.f = Ne_rpm;  % rpm
% % p2.f = VSpeed * 60/2/pi * FR * GR / Rw;  % rpm
% 
% p1.f = 2*pi/60 * Ne_rpm;  % rad/s
% p2.f = VSpeed * FR * GR / Rw;  % rad/s
% 
% 
% 
% if p1.f==0
%     w_ratio = p2.f/0.1;
% else
%     w_ratio = p2.f/p1.f;
% end
% 
% %  convert speed ratio to capacity factor
% thresh1 = 0.99;
% thresh2 = 1.07;
% thresh3 = 0.85;
% a1 = 11;
% a2 = -10.4038;
% a3 = -1.2657862;
% a4 = 0.28137862;
% a5 = 30.9091;
% a6 = 11118.1;
% a7 = 7.22274;
% a8 = -1.10485;
% a9 = -0.102677;
% b1 = 2.1  ;
% b2 = 1.30588 ;
% b3 = 0.99;
% 
% if (w_ratio < thresh1) 
%     kappa = ((a1 + a2 * w_ratio) / (1 + a3 * w_ratio + a4 * w_ratio^2));
% else
%     if (w_ratio < thresh2) 
%         kappa = (a5 + (w_ratio-thresh1)*a6);
%     else
%         kappa = (a7 / (1 + a8 * exp(a9 * w_ratio)));
%     end
% end
% 
% %  convert speed ratio to torque ratio
% if (w_ratio < thresh3) 
%     torque_ratio = (b1 - b2 * w_ratio);
% else
%     torque_ratio = b3;
% end                                                      
%     kappa = kappa/2; % tune the parameters
%     
% 	p1.e = (p1.f/kappa)^2*sign(1-w_ratio);
% 	p2.e = torque_ratio*p1.e;
%     
%     F_tract = p2.e * effi_trnsmtn * GR * FR / Rw; 
% outspeed = p2.f;
%     % EngineTorque - p1.e = J_Eng * d_w_Eng
%     d_Ne = (EngineTorque - p1.e)/J_Eng * 60/2/pi;
% %     if EngineTorque>100
% %         [EngineTorque, p1.e]
% %     end
% end
%%%%%%%%%%%%%%%%%%%%%%%%%%%%%%%%%%%%%%%%%%%%%%%%%

% 
% 
% function [d_Ne,F_tract,outspeed,w_ratio]  = gearbox_control(Ne_rpm, VSpeed, GearLevel, EngineTorque)
% %#codegen
% % Ne_rpm [rpm]
% % VSpeed [m/s]
% % GearLevel [1~6]
% % EngineTorque [Nm]
% % F_tract [N]
% % d_Ne [rpm]
% p1.e =0;
% p2.e =0;
% p1.f =0;
% p2.f =0;
% 
% 
% % parameters:
% gearRatio = [3.97	2.31	1.51	1.14	0.85	0.67]';
% FR = 3.51;  % checked with Rasoul 0802
% Rw      = 0.41;     % Tire radius [m] changed  % to match engine speed during 200-300s
% effi_trnsmtn = 0.9;
% J_Eng = 1.53; %  guess. [kg*m^2]
% 
% GR = gearRatio(GearLevel);  
% 
% % ??????? rpm or rad/s?
% p1.f = Ne_rpm;  % rpm
% p2.f = VSpeed * 60/2/pi * FR * GR / Rw;  % rpm
% 
% p1.f = 2*pi/60 * Ne_rpm;  % rad/s
% p2.f = VSpeed * FR * GR / Rw;  % rad/s
% 
% 
% 
% if p1.f==0
%     w_ratio = p2.f/0.1;
% else
%     w_ratio = p2.f/p1.f;
% end;
% 
% %  convert speed ratio to capacity factor
% % Original Tulga and Xinyi's parameters
% % thresh1 = 0.99;
% % thresh2 = 1.07;
% % thresh3 = 0.85;
% % a1 = 11;
% % a2 = -10.4038;
% % a25 = 0;
% % a3 = -1.2657862;
% % a4 = 0.28137862;
% % a5 = 30.9091;
% % a6 = 11118.1;
% % a7 = 7.22274;
% % a8 = -1.10485;
% % a9 = -0.102677;
% % b1 = 2.1;
% % b2 = 1.30588;
% % b3 = 0.99;
% % TuneRatio = 1;
% 
% % parameters from shape in reference:
% % Nonlinear Robust Control of Torque Converter
% % Clutch Slip System for Passenger Vehicles Using
% % Advanced Torque Estimation Algorithms
% thresh1 = 1;
% thresh2 = 1.07;
% thresh3 = 0.85;
% a1 = 11;
% a2 = -10.4038/1.2;
% a25 = 0;
% a3 = -1.2657862;
% a4 = 0.28137862;
% a5 = 30.9091/43*202;
% a6 = 11118.1;
% a7 = 7.22274*150*2.5/9;
% a8 = -1.10485;
% a9 = -0.102677*4.5;
% b1 = 2.1;
% b2 = 1.30588;
% b3 = 0.99;
% 
% 
% TuneRatio = 2;
% 
% if (w_ratio < thresh1) 
%     kappa = ((a1 + a2 * w_ratio + a25* w_ratio^2) /(1 + a3 * w_ratio + a4 * w_ratio^2));
% else
%     if (w_ratio < thresh2) 
%         kappa = (a5 + (w_ratio-thresh1)*a6);
%     else
%         kappa = 1/sqrt((1/11^2-1/923^2)/4/(1.5-1.07)*(w_ratio-thresh2)+1/923^2);
%         % kappa = (a7 / (1 + a8 * exp(a9 * w_ratio)));
%     end
% end
% kappa = kappa/TuneRatio; % tune the parameters
% %  convert speed ratio to torque ratio
% % 	if (w_ratio < thresh3) 
% % 		torque_ratio = (b1 - b2 * w_ratio);
% % 	else
% % 		torque_ratio = b3;
% %     end                                                     
%     if (w_ratio < thresh3) 
%         torque_ratio = (b1 - b2 * w_ratio);
%     elseif w_ratio >= thresh3 && w_ratio<=1
%         torque_ratio = b3;
%     else
%         torque_ratio = b3 + w_ratio-1;
%     end
% 	p1.e = (p1.f/kappa)^2*sign(1-w_ratio);
% 	p2.e = torque_ratio*p1.e;
%     
%     F_tract = p2.e * effi_trnsmtn * GR * FR / Rw; 
% 
%     % EngineTorque - p1.e = J_Eng * d_w_Eng
%     d_Ne = (EngineTorque - p1.e)/J_Eng * 60/2/pi;
% outspeed = p2.f;
% end
% % 

%%%%%%%%%%%%%%%%%%%%%%%%%%%%%%%%%%%%%%%%%%%%%%%%%%%%%%

function [d_Ne,F_tract,outspeed,w_ratio,p_1_e,p_2_e,GR]  = gearbox_control(time_now, time_start, Ne_rpm, VSpeed, last_gearlevel, GearLevel, EngineTorque, last_p_2_f, d_Ne_in)
%#codegen
% Ne_rpm [rpm]
% VSpeed [m/s]
% GearLevel [1~6]
% EngineTorque [Nm]
% F_tract [N]
% d_Ne [rpm]
p1.e =0;
p2.e =0;
p1.f =0;
p2.f =0;


% parameters:
gearRatio = [3.97	2.31	1.51	1.14	0.85	0.67]';
FR = 3.51;  % checked with Rasoul 0802
Rw      = 0.41;     % Tire radius [m] changed  % to match engine speed during 200-300s
effi_trnsmtn = 0.9;
J_Eng = 1.53; % Original value when doing alpha openloop: 1.53; %  guess. [kg*m^2]
%time_duration = [0.9,0.9,0.8,0.7,0.7,0.7];   % 0.5 [s] gear shift duration.
time_duration = [0.7,0.7,0.6,0.5,0.5,0.5];   % 0.5 [s] gear shift duration.

% ---------------------------------------------
% This part modified based on Tulga's code:
% ng = gr2 + ((gr1-gr2)/dur)*(time-ts);
% nt = gr2*eff2 + ((gr1*eff1-gr2*eff2)/dur)*(time-ts);
if time_now < time_start + time_duration(GearLevel)
    ratio = (time_now - time_start)/time_duration(GearLevel);
    GR = gearRatio(GearLevel) * ratio + gearRatio(last_gearlevel) * (1 - ratio);  
else
    GR = gearRatio(GearLevel);
end
% ---------------------------------------------

% ??????? rpm or rad/s?
p1.f = Ne_rpm;  % rpm
p2.f = VSpeed * 60/2/pi * FR * GR / Rw;  % rpm

p1.f = 2*pi/60 * Ne_rpm;  % rad/s
p2.f = VSpeed * FR * GR / Rw;  % rad/s
% p2.f = max(min(p2.f, last_p_2_f+80*0.02), last_p_2_f-80*0.02); % Removed
% because already done the smoothing in GR. This line generates similar Ne
% and slightly less torque than if using linear combination above. 


if p1.f<=0.1
    w_ratio = p2.f/0.1;
else
    w_ratio = p2.f/p1.f;
end

%  convert speed ratio to capacity factor

thresh1 = 1;
thresh2 = 1.07;
thresh3 = 0.85;
a1 = 11.5;
a2 = -10.4038/1.2;
a25 = -0.04;
a3 = -1.2657862;
a4 = 0.28137862;
a5 = 30.9091/43*202;
a6 = 11118.1;
a7 = 7.22274*150*2.5/9;
a8 = -1.10485;
a9 = -0.102677*4.5;
b1 = 2.1;
b2 = 1.30588;
b3 = 0.99;
TuneRatio = 2;

% b1 = 1.6;
% b2 = 0.90588;

if (w_ratio <= thresh1) 
    if  w_ratio >0.5
        % xx=interp1([0.5,0.6,0.7,0.8,0.9,1],[0.9,0.85,0.7,0.6,0.3,0.01],w_ratio,'PCHIP');
        xx=interp1([0.5,0.6,0.7,0.8,0.9,1],[0.85,0.78,0.65,0.5,0.3,0.01],w_ratio,'PCHIP');
        xx = max(xx,0);
        kappa = sqrt(1/xx/0.033)*TuneRatio;
        
    else
        % xx=interp1([0,0.4,0.5],[1,0.95,0.9],w_ratio,'PCHIP');
        xx=interp1([0,0.4,0.5],[1,0.9,0.85],w_ratio,'PCHIP');
        xx = max(xx,0);
        kappa = sqrt(1/xx/0.033)*TuneRatio;
        
    end
else
    if (w_ratio < thresh2) 
        kappa = (a5 + (w_ratio-thresh1)*a6);
    else
        kappa = (1/sqrt((1/11^2-1/923^2)/4/(1.5-1.07)*(w_ratio-thresh2)+1/923^2))*1.0;
        % kappa = ((a7+(exp(w_ratio))^-2-2) / (1 + a8 * exp(a9 * w_ratio)))+1/(10^20*(25*(w_ratio-thresh2)+0.1).^20);
    end
end

if (w_ratio < thresh3) 
    torque_ratio = (b1 - b2 * w_ratio);
elseif (w_ratio >= thresh3) && (w_ratio<=1)
    torque_ratio = b3;
else
    torque_ratio = b3 + (w_ratio-1)*2;
    torque_ratio = b3 + (w_ratio-1)*1 + 2*((1-1.5)^2-(w_ratio-1.5)^2);
    
    % torque_ratio = b3 + w_ratio-1;
end
kappa = kappa/TuneRatio; % tune the parameters

	p1.e = (p1.f/kappa)^2*sign(1-w_ratio);
	p2.e = torque_ratio*p1.e;
    
    F_tract = p2.e * effi_trnsmtn * GR * FR / Rw; 

    % EngineTorque - p1.e = J_Eng * d_w_Eng
    d_Ne = (EngineTorque - p1.e - 0.0*d_Ne_in)/J_Eng * 60/2/pi;
    
    p_1_e = p1.e;
    p_2_e = p2.e;
    
outspeed = p2.f;
end
